simulink model "LoFT_Example1"  (R2022b)
settings: Solver=ode4  StartTime=0.0  StopTime=500  FixedStep=simu.dt  RelTol=1e-3
PreLoadFcn:
  | simu.dt = 0.0125;
  | simu.Tmax = 600;
undefined symbols (not defined in the file): body, circtime, Communication, irkb, LoFT, Turbwind, waves, wind
libraries: simulink x25
(part 4 of 4)

== system LoFT_Example1/FOWT System/FOWT3/Aerodynamics and Local Control Systems/Local Control Systems/Subsystem1/Gain Scheduling ==
  In1 : Inport
  In3 : Inport  Port=2
  In2 : Inport  Port=3
  1-D Lookup Table1 : Lookup_n-D  NumberOfTableDimensions=1  BreakpointsForDimension1=Controller.R.PC_GS_angles  Table=Controller.R.PC_GS_KI  InternalRulePriority=Speed  RndMeth=Simplest
  1-D Lookup Table2 : Lookup_n-D  NumberOfTableDimensions=1  BreakpointsForDimension1=Controller.R.PC_GS_angles  Table=Controller.R.PC_GS_KP  InternalRulePriority=Speed  RndMeth=Simplest
  Add : Sum
  Add1 : Sum
  Constant1 : Constant  Value=90*pi/180
  Delay : Delay  DelayLength=1  InitialCondition=0
  Gain : Gain  Gain=simu.dt
  Product : Product
  Product1 : Product
  Saturation Dynamic : simulink/Discontinuities/Saturation Dynamic  OutMin=[]  OutMax=[]  OutDataTypeStr=Inherit: Same as second input  OutDataType=fixdt(1, 16)  OutScaling=2^-10  DoSatur=off
  Saturation1 : Saturate  UpperLimit=Controller.R.PC_GS_KI(end)  LowerLimit=Controller.R.PC_GS_KI(1)
  Saturation3 : Saturate  UpperLimit=Controller.R.PC_GS_KP(end)  LowerLimit=Controller.R.PC_GS_KP(1)
  Out1 : Outport
  wires:
  Product/1 -> Add1/1
  Add1/1 -> Out1/1
  Delay/1 -> Add/2
  Saturation Dynamic/1 -> Delay/1, Add1/2
  Constant1/1 -> Saturation Dynamic/1
  In3/1 -> Saturation Dynamic/3
  Add/1 -> Saturation Dynamic/2
  Gain/1 -> Add/1
  Product1/1 -> Gain/1
  Saturation1/1 -> Product1/2
  Saturation3/1 -> Product/2
  In1/1 -> Product1/1, Product/1
  In2/1 -> 1-D Lookup Table2/1, 1-D Lookup Table1/1
  1-D Lookup Table2/1 -> Saturation3/1
  1-D Lookup Table1/1 -> Saturation1/1

== system LoFT_Example1/FOWT System/FOWT4/Aerodynamics and Local Control Systems/Local Control Systems/Subsystem1/Gain Scheduling ==
  In1 : Inport
  In3 : Inport  Port=2
  In2 : Inport  Port=3
  1-D Lookup Table1 : Lookup_n-D  NumberOfTableDimensions=1  BreakpointsForDimension1=Controller.R.PC_GS_angles  Table=Controller.R.PC_GS_KI  InternalRulePriority=Speed  RndMeth=Simplest
  1-D Lookup Table2 : Lookup_n-D  NumberOfTableDimensions=1  BreakpointsForDimension1=Controller.R.PC_GS_angles  Table=Controller.R.PC_GS_KP  InternalRulePriority=Speed  RndMeth=Simplest
  Add : Sum
  Add1 : Sum
  Constant1 : Constant  Value=90*pi/180
  Delay : Delay  DelayLength=1  InitialCondition=0
  Gain : Gain  Gain=simu.dt
  Product : Product
  Product1 : Product
  Saturation Dynamic : simulink/Discontinuities/Saturation Dynamic  OutMin=[]  OutMax=[]  OutDataTypeStr=Inherit: Same as second input  OutDataType=fixdt(1, 16)  OutScaling=2^-10  DoSatur=off
  Saturation1 : Saturate  UpperLimit=Controller.R.PC_GS_KI(end)  LowerLimit=Controller.R.PC_GS_KI(1)
  Saturation3 : Saturate  UpperLimit=Controller.R.PC_GS_KP(end)  LowerLimit=Controller.R.PC_GS_KP(1)
  Out1 : Outport
  wires:
  1-D Lookup Table1/1 -> Saturation1/1
  1-D Lookup Table2/1 -> Saturation3/1
  In2/1 -> 1-D Lookup Table1/1, 1-D Lookup Table2/1
  In1/1 -> Product/1, Product1/1
  Saturation3/1 -> Product/2
  Saturation1/1 -> Product1/2
  Product1/1 -> Gain/1
  Gain/1 -> Add/1
  Add/1 -> Saturation Dynamic/2
  In3/1 -> Saturation Dynamic/3
  Constant1/1 -> Saturation Dynamic/1
  Saturation Dynamic/1 -> Add1/2, Delay/1
  Delay/1 -> Add/2
  Add1/1 -> Out1/1
  Product/1 -> Add1/1

== system LoFT_Example1/FOWT System/FOWT5/Aerodynamics and Local Control Systems/Local Control Systems/Subsystem1/Gain Scheduling ==
  In1 : Inport
  In3 : Inport  Port=2
  In2 : Inport  Port=3
  1-D Lookup Table1 : Lookup_n-D  NumberOfTableDimensions=1  BreakpointsForDimension1=Controller.R.PC_GS_angles  Table=Controller.R.PC_GS_KI  InternalRulePriority=Speed  RndMeth=Simplest
  1-D Lookup Table2 : Lookup_n-D  NumberOfTableDimensions=1  BreakpointsForDimension1=Controller.R.PC_GS_angles  Table=Controller.R.PC_GS_KP  InternalRulePriority=Speed  RndMeth=Simplest
  Add : Sum
  Add1 : Sum
  Constant1 : Constant  Value=90*pi/180
  Delay : Delay  DelayLength=1  InitialCondition=0
  Gain : Gain  Gain=simu.dt
  Product : Product
  Product1 : Product
  Saturation Dynamic : simulink/Discontinuities/Saturation Dynamic  OutMin=[]  OutMax=[]  OutDataTypeStr=Inherit: Same as second input  OutDataType=fixdt(1, 16)  OutScaling=2^-10  DoSatur=off
  Saturation1 : Saturate  UpperLimit=Controller.R.PC_GS_KI(end)  LowerLimit=Controller.R.PC_GS_KI(1)
  Saturation3 : Saturate  UpperLimit=Controller.R.PC_GS_KP(end)  LowerLimit=Controller.R.PC_GS_KP(1)
  Out1 : Outport
  wires:
  Product/1 -> Add1/1
  Add1/1 -> Out1/1
  Delay/1 -> Add/2
  Saturation Dynamic/1 -> Delay/1, Add1/2
  Constant1/1 -> Saturation Dynamic/1
  In3/1 -> Saturation Dynamic/3
  Add/1 -> Saturation Dynamic/2
  Gain/1 -> Add/1
  Product1/1 -> Gain/1
  Saturation1/1 -> Product1/2
  Saturation3/1 -> Product/2
  In1/1 -> Product1/1, Product/1
  In2/1 -> 1-D Lookup Table2/1, 1-D Lookup Table1/1
  1-D Lookup Table2/1 -> Saturation3/1
  1-D Lookup Table1/1 -> Saturation1/1

== matlab function LoFT_Example1/FOWT System/FOWT5/Hydrodynamics/radiation force/MATLAB Function ==
  data: velocity input; radiationdamping output; irkb input; circtime input
function radiationdamping  = fcn(velocity,irkb,circtime)

radiationdamping  = ConvolutionIntegral_interp(velocity,irkb,circtime);
end

== matlab function LoFT_Example1/FOWT System/FOWT1/Hydrodynamics/excitation force/WECSim Linear wave excitiation ==
  data: A input; Fext output; w input; fExtRE input; fExtIM input; phaseRand input; dw input; time input; WaveDir input; spread input; fExtMD input
function Fext = irregExcF(A,w,fExtRE,fExtIM,phaseRand,dw,time,WaveDir,spread,fExtMD)

Fext = irregExcF(A,w,fExtRE,fExtIM,phaseRand,dw,time,WaveDir,spread,fExtMD);

end

== matlab function LoFT_Example1/FOWT System/FOWT1/Hydrodynamics/radiation force/MATLAB Function ==
  data: velocity input; radiationdamping output; irkb input; circtime input
function radiationdamping  = fcn(velocity,irkb,circtime)

radiationdamping  = ConvolutionIntegral_interp(velocity,irkb,circtime);
end

== matlab function LoFT_Example1/FOWT System/FOWT2/Hydrodynamics/excitation force/WECSim Linear wave excitiation ==
  data: A input; Fext output; w input; fExtRE input; fExtIM input; phaseRand input; dw input; time input; WaveDir input; spread input; fExtMD input
function Fext = irregExcF(A,w,fExtRE,fExtIM,phaseRand,dw,time,WaveDir,spread,fExtMD)

Fext = irregExcF(A,w,fExtRE,fExtIM,phaseRand,dw,time,WaveDir,spread,fExtMD);

end

== matlab function LoFT_Example1/FOWT System/FOWT2/Hydrodynamics/radiation force/MATLAB Function ==
  data: velocity input; radiationdamping output; irkb input; circtime input
function radiationdamping  = fcn(velocity,irkb,circtime)

radiationdamping  = ConvolutionIntegral_interp(velocity,irkb,circtime);
end

== matlab function LoFT_Example1/FOWT System/FOWT3/Hydrodynamics/excitation force/WECSim Linear wave excitiation ==
  data: A input; Fext output; w input; fExtRE input; fExtIM input; phaseRand input; dw input; time input; WaveDir input; spread input; fExtMD input
function Fext = irregExcF(A,w,fExtRE,fExtIM,phaseRand,dw,time,WaveDir,spread,fExtMD)

Fext = irregExcF(A,w,fExtRE,fExtIM,phaseRand,dw,time,WaveDir,spread,fExtMD);

end

== matlab function LoFT_Example1/FOWT System/FOWT3/Hydrodynamics/radiation force/MATLAB Function ==
  data: velocity input; radiationdamping output; irkb input; circtime input
function radiationdamping  = fcn(velocity,irkb,circtime)

radiationdamping  = ConvolutionIntegral_interp(velocity,irkb,circtime);
end

== matlab function LoFT_Example1/FOWT System/FOWT4/Hydrodynamics/excitation force/WECSim Linear wave excitiation ==
  data: A input; Fext output; w input; fExtRE input; fExtIM input; phaseRand input; dw input; time input; WaveDir input; spread input; fExtMD input
function Fext = irregExcF(A,w,fExtRE,fExtIM,phaseRand,dw,time,WaveDir,spread,fExtMD)

Fext = irregExcF(A,w,fExtRE,fExtIM,phaseRand,dw,time,WaveDir,spread,fExtMD);

end

== matlab function LoFT_Example1/FOWT System/FOWT4/Hydrodynamics/radiation force/MATLAB Function ==
  data: velocity input; radiationdamping output; irkb input; circtime input
function radiationdamping  = fcn(velocity,irkb,circtime)

radiationdamping  = ConvolutionIntegral_interp(velocity,irkb,circtime);
end

== matlab function LoFT_Example1/FOWT System/FOWT5/Hydrodynamics/excitation force/WECSim Linear wave excitiation ==
  data: A input; Fext output; w input; fExtRE input; fExtIM input; phaseRand input; dw input; time input; WaveDir input; spread input; fExtMD input
function Fext = irregExcF(A,w,fExtRE,fExtIM,phaseRand,dw,time,WaveDir,spread,fExtMD)

Fext = irregExcF(A,w,fExtRE,fExtIM,phaseRand,dw,time,WaveDir,spread,fExtMD);

end
